simulink model "Project1_Part2_Option3_MODEL"  (R2023b)
settings: Solver=VariableStepAuto  StartTime=0.0  StopTime=25  RelTol=1e-3
values from neighbouring files (symbols this model uses):
  A = T_0_values(l)    [Project1_Part2.m]    (also in Project1_Part2_Option1_CODE.m = A_values(j); Project1_Part2_Option2_CODE.m = A_values(j); Project1_Part2_Option3_CODE.m = A_values(j))
  b1 = 1    [Project1_Part2.m]    (also in Project1_Part2_Option1_CODE.m; Project1_Part2_Option2_CODE.m; Project1_Part2_Option3_CODE.m)
  b2 = 1    [Project1_Part2.m]    (also in Project1_Part2_Option1_CODE.m; Project1_Part2_Option2_CODE.m; Project1_Part2_Option3_CODE.m)
  J1 = 100    [Project1_Part2.m]    (also in Project1_Part2_Option1_CODE.m; Project1_Part2_Option2_CODE.m; Project1_Part2_Option3_CODE.m)
  J2 = 1    [Project1_Part2.m]    (also in Project1_Part2_Option1_CODE.m; Project1_Part2_Option2_CODE.m; Project1_Part2_Option3_CODE.m)
settings Model: Creator=turtl  LastModifiedBy=turtl

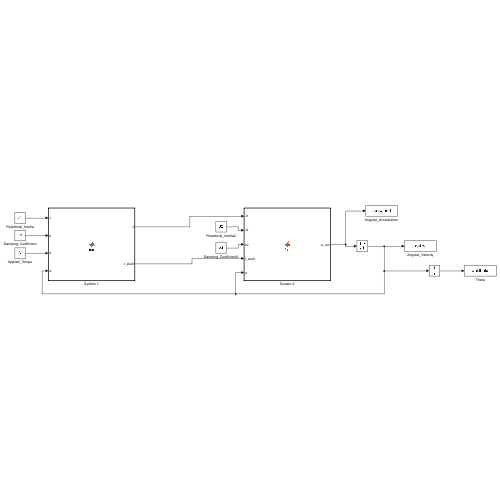
[thumbnail: Simulink's stored preview of the top-level diagram]
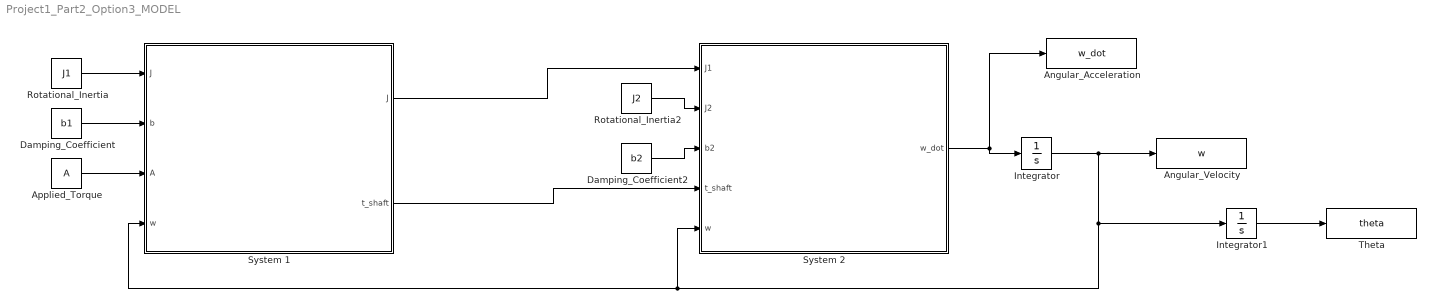
== system Project1_Part2_Option3_MODEL ==
  Angular_Acceleration : ToWorkspace  VariableName=w_dot  SaveFormat=Timeseries  SampleTime=-1
  Angular_Velocity : ToWorkspace  VariableName=w  SaveFormat=Timeseries  SampleTime=-1
  Applied_Torque : Constant  Value=A
  Damping_Coefficient : Constant  Value=b1
  Damping_Coefficient2 : Constant  Value=b2
  Integrator : Integrator  LimitOutput=on  UpperSaturationLimit=10000  LowerSaturationLimit=0
  Integrator1 : Integrator
  Rotational_Inertia : Constant  Value=J1
  Rotational_Inertia2 : Constant  Value=J2
  System 1 : MATLAB Function  TreatAsAtomicUnit=on
  System 2 : MATLAB Function  TreatAsAtomicUnit=on
  Theta : ToWorkspace  VariableName=theta  SaveFormat=Timeseries  SampleTime=-1
  wires:
  Damping_Coefficient2/1 -> System 2/3(b2)
  Integrator1/1 -> Theta/1
  System 2/1(w_dot) -> Angular_Acceleration/1, Integrator/1
  Integrator/1 -> Angular_Velocity/1, Integrator1/1, System 2/5(w), System 1/4(w)
  Applied_Torque/1 -> System 1/3(A)
  Rotational_Inertia/1 -> System 1/1("J ")
  Damping_Coefficient/1 -> System 1/2(b)
  Rotational_Inertia2/1 -> System 2/2(J2)
  System 1/2(t_shaft) -> System 2/4(t_shaft)
  System 1/1(J) -> System 2/1(J1)

== matlab function Project1_Part2_Option3_MODEL/System 1 ==
  data: J input; J output; b input; A input; w input; t_shaft output
function [J,t_shaft] = fcn(J,b,A,w)
t_shaft = A-b*w;
end

== matlab function Project1_Part2_Option3_MODEL/System 2 ==
  data: J1 input; w_dot output; J2 input; b2 input; t_shaft input; w input
function w_dot = fcn(J1,J2,b2, t_shaft,w)
w_dot = (1/(J1+J2))*(t_shaft-b2*w);
end
